simulink model "servoNonLinearSimObserved"  (R2022b)
settings: Solver=VariableStepAuto  StartTime=0.0  StopTime=15  RelTol=10e-8
settings Model: Creator=HP  LastModifiedBy=HP
settings SolverCC: AlgebraicLoopSolver=TrustRegion
settings DebuggingCC: UnconnectedInputMsg=warning  UnconnectedOutputMsg=warning  UnconnectedLineMsg=warning  SFMachineParentedDataDiag=warning
settings ModelReferenceCC: EnableRefExpFcnMdlSchedulingChecks=on
settings RTWCC: DLArmComputeVersion=19.05

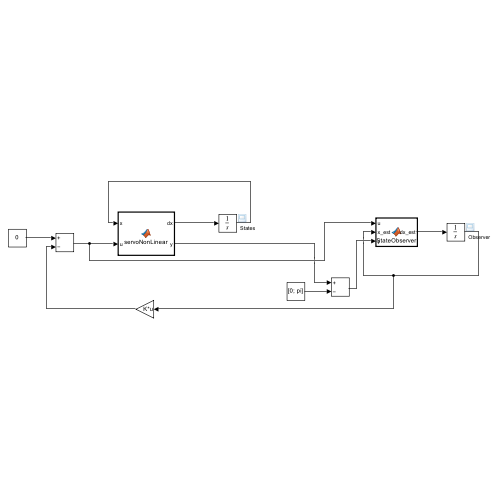
[thumbnail: Simulink's stored preview of the top-level diagram]
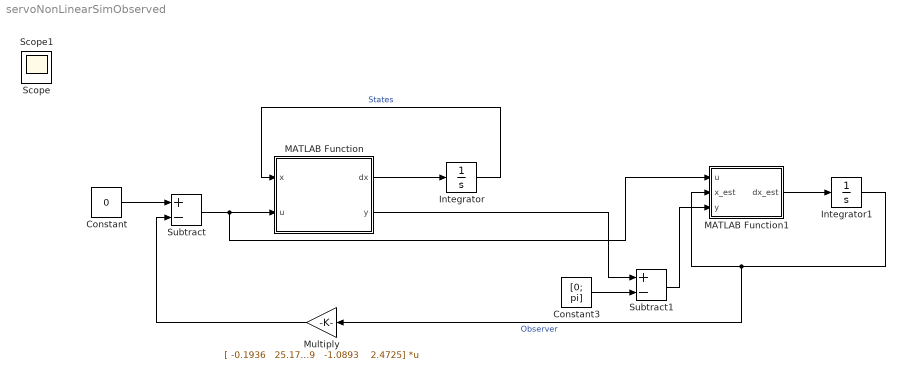
== system servoNonLinearSimObserved ==
  Constant : Constant  Value=0
  Constant3 : Constant  Value=[0; pi]
  Integrator : Integrator  InitialCondition=[0; pi-pi/10; 0; 0]  IgnoreLimit=on
  Integrator1 : Integrator  InitialCondition=[0; -pi/10; 0; 0]
  MATLAB Function : MATLAB Function  TreatAsAtomicUnit=on
  MATLAB Function1 : MATLAB Function  TreatAsAtomicUnit=on
  Multiply : Gain  Gain="[ -0.1936   25.1799   -1.0893    2.4725]"  Multiplication=Matrix(K*u)
  Subtract : Sum  Inputs=+-
  Subtract1 : Sum  Inputs=+-
  Scope : Scope
  Scope1 : Scope
  wires:
  MATLAB Function/1(dx) -> Integrator/1
  Integrator/1 -> MATLAB Function/1(x)  "States"
  Multiply/1 -> Subtract/2
  Constant/1 -> Subtract/1
  Subtract/1 -> MATLAB Function1/1(u), MATLAB Function/2(u)
  Constant3/1 -> Subtract1/2
  MATLAB Function/2(y) -> Subtract1/1
  Subtract1/1 -> MATLAB Function1/3(y)
  MATLAB Function1/1(dx_est) -> Integrator1/1
  Integrator1/1 -> MATLAB Function1/2(x_est), Multiply/1  "Observer"

== matlab function servoNonLinearSimObserved/MATLAB Function ==
  data: x input; u input; dx output; y output
function [dx,y] = servoNonLinear(x,u)
%% Motor
% Resistance
Rm = 8.4;
% Current-torque (N-m/A)
kt = 0.042;
% Back-emf constant (V-s/rad)
km = 0.042;
%
%% Rotary Arm
% Mass (kg)
mr = 0.095;
% Total length (m)
r = 0.085;
% Moment of inertia about pivot (kg-m^2)
Jr = mr*r^2/3;
% Equivalent Viscous Damping Coefficient (N-m-s/rad)
br = 1e-3; % damping tuned heuristically to match QUBE-Sero 2 response
%
%% Pendulum Link
% Mass (kg)
mp = 0.024;
% Total length (m)
Lp = 0.129;
% Pendulum center of mass (m)
l = Lp/2;
% Moment of inertia about pivot (kg-m^2)
Jp = mp*Lp^2/3;
% Equivalent Viscous Damping Coefficient (N-m-s/rad)
bp = 5e-5; % damping tuned heuristically to match QUBE-Sero 2 response
% Gravity Constant
g = 9.81;
Jt=Jp*Jr-mp^2*l^2*r^2;

%Nonlinear system 
theta=x(1);
alpha=x(2);
theta2=x(3);
alpha2=x(4);
Tau=u;
dtheta2=(Jp*Tau - Jp*br*theta2 - 2*Jp^2*alpha2*theta2*cos(alpha)*sin(alpha) + alpha2*bp*l*mp*r*cos(alpha) + g*l^2*mp^2*r*cos(alpha)*sin(alpha) + Jp*alpha2^2*l*mp*r*sin(alpha) - Jp*l*mp*r*theta2^2*cos(alpha)^2*sin(alpha))/(Jp^2*sin(alpha)^2 + Jr*Jp - l^2*mp^2*r^2*cos(alpha)^2);
dalpha2=-(Jr*alpha2*bp + Jp*alpha2*bp*sin(alpha)^2 - Jp^2*theta2^2*cos(alpha)*sin(alpha)^3 + Jp*g*l*mp*sin(alpha)^3 - Jp*Jr*theta2^2*cos(alpha)*sin(alpha) + Jr*g*l*mp*sin(alpha) + Tau*l*mp*r*cos(alpha) + alpha2^2*l^2*mp^2*r^2*cos(alpha)*sin(alpha) - br*l*mp*r*theta2*cos(alpha) - 2*Jp*alpha2*l*mp*r*theta2*cos(alpha)^2*sin(alpha))/(Jp^2*sin(alpha)^2 + Jr*Jp - l^2*mp^2*r^2*cos(alpha)^2);
dx=x;
dx(1)=theta2;
dx(2)=alpha2;
dx(3)=dtheta2;
dx(4)=dalpha2;
y=[0;0];
y(1)=theta;
y(2)=alpha;

== matlab function servoNonLinearSimObserved/MATLAB Function1 ==
  data: u input; dx_est output; x_est input; y input
function dx_est  = StateObserver(u,x_est,y)
F = [-13.6162    0.5990    1.0000         0;
     3.8834  -25.3861         0    1.0000;
    -3.7884    7.8602  -10.1274   -0.5005;
    54.6516 -155.1368  -10.0097   -0.8702];


B=[ 0;
    0;
    10127.4369;
    10009.6760];

L= [13.6162   -0.5990;
   -3.8834   25.3861;
    3.7884  144.1456;
  -54.6516  419.4448];

dx_est=F*x_est+L*y+B*u;
